simulink model "ControlSystemLoadChange"  (R2023a)
settings: Solver=VariableStepAuto  StartTime=0.0  StopTime=3.0  RelTol=1e-3
undefined symbols (not defined in the file): ADC, B, DutyC, FV, GR, J, K, Ki, Kp, L, R, RH, Ti, Vbat
settings Model: Creator=NG22  LastModifiedBy=NG22

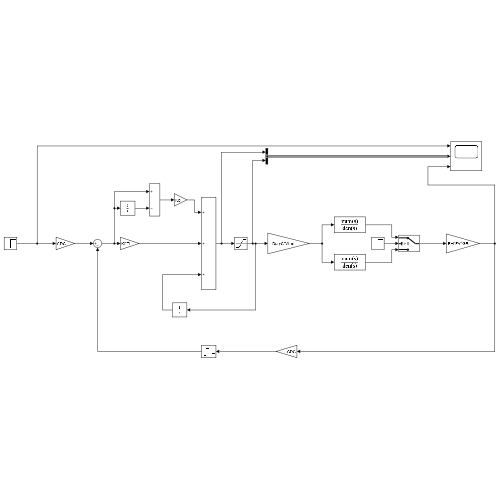
[thumbnail: Simulink's stored preview of the top-level diagram]
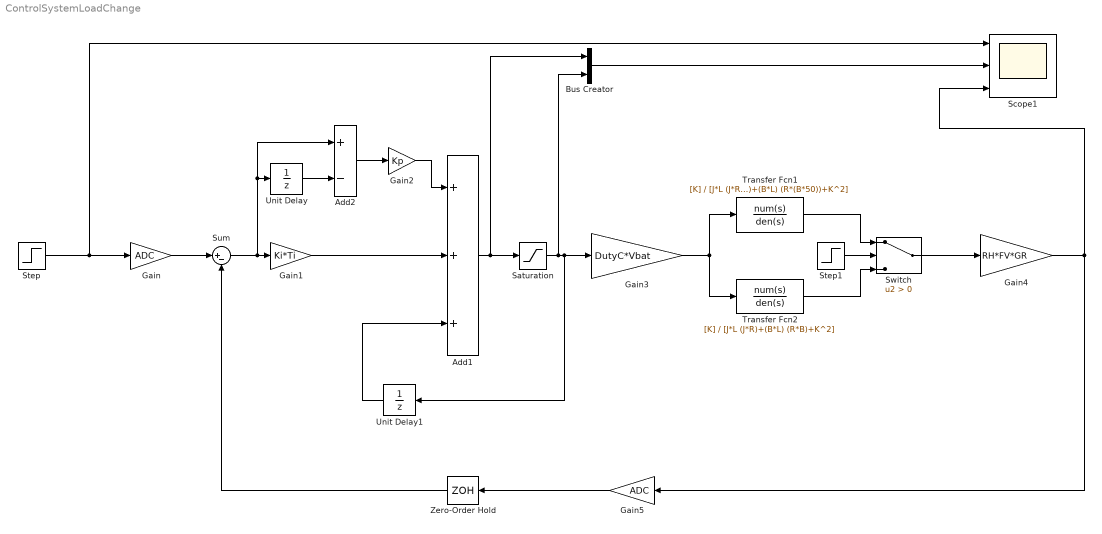
== system ControlSystemLoadChange ==
  Add1 : Sum  Inputs=+++
  Add2 : Sum  Inputs=+-
  Bus Creator : BusCreator  Inputs=2
  Gain : Gain  Gain=ADC
  Gain1 : Gain  Gain=Ki*Ti
  Gain2 : Gain  Gain=Kp
  Gain3 : Gain  Gain=DutyC*Vbat
  Gain4 : Gain  Gain=RH*FV*GR
  Gain5 : Gain  Gain=ADC
  Saturation : Saturate
  Scope1 : Scope  NumInputPorts=3
  Step : Step  SampleTime=0
  Step1 : Step  Time=2  SampleTime=0
  Sum : Sum  Inputs=|+-
  Switch : Switch  Criteria=u2 > Threshold  SaturateOnIntegerOverflow=off  InputSameDT=off
  Transfer Fcn1 : TransferFcn  Numerator=[K]  Denominator=[J*L (J*R)+(B*L) (R*(B*50))+K^2]
  Transfer Fcn2 : TransferFcn  Numerator=[K]  Denominator=[J*L (J*R)+(B*L) (R*B)+K^2]
  Unit Delay : UnitDelay  SampleTime=-1  HasFrameUpgradeWarning=on
  Unit Delay1 : UnitDelay  SampleTime=-1  HasFrameUpgradeWarning=on
  Zero-Order Hold : ZeroOrderHold  SampleTime=-1
  wires:
  Step/1 -> Scope1/1, Gain/1
  Gain/1 -> Sum/1
  Sum/1 -> Gain1/1, Unit Delay/1, Add2/1
  Unit Delay/1 -> Add2/2
  Add2/1 -> Gain2/1
  Gain2/1 -> Add1/1
  Unit Delay1/1 -> Add1/3
  Saturation/1 -> Unit Delay1/1, Gain3/1, Bus Creator/2
  Add1/1 -> Bus Creator/1, Saturation/1
  Bus Creator/1 -> Scope1/2
  Gain4/1 -> Gain5/1, Scope1/3
  Gain5/1 -> Zero-Order Hold/1
  Zero-Order Hold/1 -> Sum/2
  Gain1/1 -> Add1/2
  Step1/1 -> Switch/2
  Gain3/1 -> Transfer Fcn2/1, Transfer Fcn1/1
  Transfer Fcn1/1 -> Switch/1
  Transfer Fcn2/1 -> Switch/3
  Switch/1 -> Gain4/1
